simulink model "P2_SIL_Model_Diag"  (R2016a)
settings: Solver=ode2  StartTime=0.0  StopTime=Cycle_End  RelTol=1e-3
undefined symbols (not defined in the file): air, APP1_OOR, APP2_OOR, APP_Conversion_IN, APP_Mismatch, bms_inletair_temp, bms_maxchargecurrent, bms_maxdischargecurrent, BMS_Notfallkuehlung, BPP_Flt, cal, clt, ClutchEngag, CrankRequest, dcdc, eng, Engine, EngOverTemp, ENGTRQ_MSMCH_Degraded_CP, ENGTRQ_MSMCH_ErrCritical_CP, ENGTRQ_MSMCH_LimpHome_CP, EngTrqMismatch, env, ess, ESS, ESSOverTemp, fd, FFD, g, gb, Grade, IMG, KeyPos_Flt, KeyPosition, lib_APP_Conversion_IN, lib_ESS_plant_V1_2, lib_OBC_Manager, LossCAN, max_vehicle_rad_air_flow, MCUOverTemp, mot, MotDirMismatch, MotOverTemp, MotTrqMismatch, mph2kph, mph2ms, NeutralGear, obc, OBC_Manager, ParkGear, PRNDL_Flt, ReverseGear, RFD, rho, ShiftLeverPosition, sigbuilder_block, Speed, t_amb, time, tloop ... (+2)
libraries: simulink x104, EC2_libraries x12, Diagnostic x11, lib_CANerror_Detect x3, Utility x1
(part 7 of 11)

== system P2_SIL_Model_Diag/Controller/HSC/Camaro Fault Detection/Signal Generator /BMS_Signals ==
  BMS_rollingAliveCnt : Subsystem
  Bus Creator : BusCreator  Inputs=9
  Constant{1..8} (8 alike) : Constant
  tag scope: BMS_Signals=global
  wires:
  Constant7/1 -> Bus Creator/4  "BMS_hvBusVolt_V"
  Bus Creator/1 -> [BMS_Signals]  "BMS_Signals"
  Constant2/1 -> Bus Creator/3  "BMS_essTemp_K"
  Constant1/1 -> Bus Creator/2  "BMS_hvBattVolt_V"
  Constant3/1 -> Bus Creator/5  "BMS_closeContactorsCmd"
  Constant4/1 -> Bus Creator/6  "BMS_contactorsClsd"
  Constant5/1 -> Bus Creator/7  "BMS_essCurr_A"
  Constant6/1 -> Bus Creator/8  "BMS_essSOC_0_1"
  Constant8/1 -> Bus Creator/9  "BMS_gdf"
  BMS_rollingAliveCnt/1(Out1) -> Bus Creator/1

== system P2_SIL_Model_Diag/Controller/HSC/Camaro Fault Detection/Signal Generator /Clutch_Signals ==
  note: LvrPosTrnsShft
      | TransEstGear
      | LockupCmd
  note: TransEstGear
      | 0 : Not Supported
      | 1 : First Gear
      | 2 : Second Gear
      | 3 : Third Gear
      | 4 : Fourth Gear
      | 5 : Fifth Gear
      | 6 : Sixth Gear
      | 7 : Seventh Gear
      | 8 : Eight Gear
      | 10: EVT Mode 1
      | 11: EVT Mode 2
      | 12: CVT Forward Gear
      | 13: Neutral Gear
      | 14: Reverse Gear
      | 15: Park Gear
  note: Lever Position:
      | 1 P
      | 2 R
      | 3 N
      | 4 D
      |
      | 1 clutch lock-up
      | 0 clutch unlock
  Bus Creator : BusCreator  Inputs=3
  Clutch_Rolling : Subsystem
  Constant : Constant
  Constant2 : Constant
  tag scope: Clutch_Signals=global
  wires:
  Constant2/1 -> Bus Creator/3  "clt_plant_spd_out"
  Constant/1 -> Bus Creator/2  "Engage_Clutch"
  Bus Creator/1 -> [Clutch_Signals]  "Clutch_Signals"
  Clutch_Rolling/1(Out1) -> Bus Creator/1

== system P2_SIL_Model_Diag/Controller/HSC/Camaro Fault Detection/Signal Generator /Driver_Signals ==
  Bus Creator1 : BusCreator  Inputs=6
  Constant{1..6} (6 alike) : Constant
  tag scope: Driver_Signals=global
  wires:
  Bus Creator1/1 -> [Driver_Signals]  "Driver_Signals"
  Constant4/1 -> Bus Creator1/2  "BPP%"
  Constant5/1 -> Bus Creator1/3  "keyPos"
  Constant3/1 -> Bus Creator1/1  "APP1%"
  Constant6/1 -> Bus Creator1/4  "APP2%"
  Constant1/1 -> Bus Creator1/5  "PRNDL"
  Constant2/1 -> Bus Creator1/6  "V [mph]"

== system P2_SIL_Model_Diag/Controller/HSC/Camaro Fault Detection/Signal Generator /ECM_Signals ==
  Bus Creator : BusCreator  Inputs=6
  Constant{1..4} (4 alike) : Constant
  ECM_CAN_Rolling : Subsystem
  EngBrkTrq[Nm] : Constant
  tag scope: ECM_Signals=global
  wires:
  Constant1/1 -> Bus Creator/2  "ECMTrqCmd[Nm]"
  Bus Creator/1 -> [ECM_Signals]  "ECM_Signals"
  Constant2/1 -> Bus Creator/3  "Engine_Speed[rpm]"
  Constant3/1 -> Bus Creator/4  "Engine_Temp[DegC]"
  Constant4/1 -> Bus Creator/5  "EngRunAtv_0_1"
  EngBrkTrq[Nm]/1 -> Bus Creator/6  "EngActStdyStTorq_Nm"
  ECM_CAN_Rolling/1(Out1) -> Bus Creator/1

== system P2_SIL_Model_Diag/Controller/HSC/Camaro Fault Detection/Signal Generator /MCU_Signals ==
  note: From sensor
  note: From sensor
  note: From sensor
  note: From HSC
  note: From Sensor
  note: Note: motor direction feedback from HSC
  note: Torque_Command from HSC
  Bus Creator : BusCreator  Inputs=10
  Constant{1..7,9..10} (9 alike) : Constant
  MCU_CAN_rolling : Subsystem
  tag scope: MCU_Signals=global
  wires:
  Constant1/1 -> Bus Creator/2  "MCUTemp_degC"
  Bus Creator/1 -> [MCU_Signals]  "MCU_Signals"
  Constant2/1 -> Bus Creator/3  "Motor_Temp_degC"
  Constant3/1 -> Bus Creator/4  "MCUTrqCmd[Nm]"
  Constant4/1 -> Bus Creator/6  "Motor_Speed[rpm]"
  Constant5/1 -> Bus Creator/7  "Direction_Command_01"
  Constant6/1 -> Bus Creator/5  "Torque_Feedback[Nm]"
  Constant7/1 -> Bus Creator/8  "Direction_Feedback"
  Constant9/1 -> Bus Creator/9  "Inverter_Enable_State"
  Constant10/1 -> Bus Creator/10  "DC_Bus_Voltage"
  MCU_CAN_rolling/1(Out1) -> Bus Creator/1

== system P2_SIL_Model_Diag/Controller/HSC/Camaro Fault Detection/Signal Generator /TCM_Signals ==
  note: Lever Position:
      | 1 P
      | 2 R
      | 3 N
      | 4 D
      |
      | 1 clutch lock-up
      | 0 clutch unlock
  note: TransEstGear calculated in TCM
      | 0 : Not Supported
      | 1 : First Gear
      | 2 : Second Gear
      | 3 : Third Gear
      | 4 : Fourth Gear
      | 5 : Fifth Gear
      | 6 : Sixth Gear
      | 7 : Seventh Gear
      | 8 : Eight Gear
      | 10: EVT Mode 1
      | 11: EVT Mode 2
      | 12: CVT Forward Gear
      | 13: Neutral Gear
      | 14: Reverse Gear
      | 15: Park Gear
  note: LvrPosTrnsShft ==PRNDL
      | TransEstGear
      | LockupCmd
  Bus Creator : BusCreator  Inputs=4
  Constant : Constant
  Constant1 : Constant
  Constant2 : Constant
  TCM_Rolling : Subsystem
  tag scope: TCM_Signals=global
  wires:
  Bus Creator/1 -> [TCM_Signals]  "TCM_Signals"
  Constant/1 -> Bus Creator/2  "LvrPosTrnsShft"
  Constant1/1 -> Bus Creator/3  "TransEstGear"
  Constant2/1 -> Bus Creator/4  "LockupCmd"
  TCM_Rolling/1(Out1) -> Bus Creator/1

== system P2_SIL_Model_Diag/Controller/HSC/Camaro Fault Detection/SystemDiag/Combined_SystemDiagnostics ==
  note: Combined_Powertrain: System Diagnostics
  In1 : Inport
  Bus Creator : BusCreator  Inputs=1
  Bus Selector : BusSelector  OutputSignals=Driver_Input_Status.Driver_Input_Status,BMS_Status.BMS_Status,MCU_Status.MCU_Status,ECM_Status.ECM_Status,TCM_CompDiag.TCM_Status,Clutch_Status.Clutch_Status
  Combined_System_Diagnostics : Stateflow chart  TreatAsAtomicUnit=on
  Override Combined_System Status : Subsystem  AncestorBlock=Diagnostic/Camaro Diagnostic/Input Conversions/DriverInput_Conversions/Override APP (%)
  Out1 : Outport
  wires:
  In1/1 -> Bus Selector/1
  Bus Creator/1 -> Out1/1  "Combined_SystemDiagOut"
  Override Combined_System Status/1(Out1) -> Bus Creator/1  "Combined_SystemStatus"
  Bus Selector/1 -> Combined_System_Diagnostics/1(Driver_Input_Status)  "<Driver_Input_Status>"
  Bus Selector/2 -> Combined_System_Diagnostics/2(BMS_Status)  "<BMS_Status>"
  Bus Selector/3 -> Combined_System_Diagnostics/3(MCU_Status)  "<MCU_Status>"
  Bus Selector/4 -> Combined_System_Diagnostics/4(ECM_Status)  "<ECM_Status>"
  Bus Selector/5 -> Combined_System_Diagnostics/5(TCM_Status)  "<TCM_Status>"
  Bus Selector/6 -> Combined_System_Diagnostics/6(Clutch_Status)  "<Clutch_Status>"
  Combined_System_Diagnostics/1(Combined_SystemStatus) -> Override Combined_System Status/1(In1)

== system P2_SIL_Model_Diag/Controller/HSC/Camaro Fault Detection/SystemDiag/eSystemDiagnostics ==
  note: BMS_Status:
      | Offline: 0
      | Limited: 1
      | Online: 2
      |
      | MCU_Status
      | Offline: 0
      | Limited: 1
      | Online :2
  note: 0: SystemStatus: Offline
      | 1: SystemStatus Limited
      | 2: SystemStatus Online
  note: eSystem: System Diagnostics
  In1 : Inport
  Bus Creator : BusCreator  Inputs=1
  Bus Selector : BusSelector  OutputSignals=BMS_Status,MCU_Status,Driver_Input_Status,TCM_Status
  Override eSystem Status : Subsystem  AncestorBlock=Diagnostic/Camaro Diagnostic/Input Conversions/DriverInput_Conversions/Override APP (%)
  To Workspace2 : ToWorkspace  VariableName=eSystemStatus  SaveFormat=Timeseries  SampleTime=-1
  eSystem_Diagnostics : Stateflow chart  TreatAsAtomicUnit=on
  Out1 : Outport
  wires:
  In1/1 -> Bus Selector/1
  Bus Selector/1 -> eSystem_Diagnostics/1(BMS_Status)  "<BMS_Status>"
  Bus Selector/2 -> eSystem_Diagnostics/2(MCU_Status)  "<MCU_Status>"
  Bus Creator/1 -> Out1/1  "eSystemDiagOut"
  Bus Selector/3 -> eSystem_Diagnostics/3(Driver_Input_Status)  "<Driver_Input_Status>"
  Override eSystem Status/1(Out1) -> To Workspace2/1, Bus Creator/1  "eSystemStatus"
  eSystem_Diagnostics/1(eSystemStatus) -> Override eSystem Status/1(In1)
  Bus Selector/4 -> eSystem_Diagnostics/4(TCM_Status)  "<TCM_Status>"

== system P2_SIL_Model_Diag/Controller/HSC/Camaro Fault Detection/SystemDiag/iceSystemDiagnostics ==
  note: iceSystem: System Diagnostics
  In1 : Inport
  Bus Creator : BusCreator  Inputs=1
  Bus Selector : BusSelector  OutputSignals=ECM_Status,Clutch_Status,TCM_Status,Driver_Input_Status
  Override iceSystem Status : Subsystem  AncestorBlock=Diagnostic/Camaro Diagnostic/Input Conversions/DriverInput_Conversions/Override APP (%)
  To Workspace2 : ToWorkspace  VariableName=iceSystemStatus  SaveFormat=Timeseries  SampleTime=-1
  iceSystem_Diagnostics : Stateflow chart  TreatAsAtomicUnit=on
  Out1 : Outport
  wires:
  Override iceSystem Status/1(Out1) -> To Workspace2/1, Bus Creator/1  "iceSystemStatus"
  Bus Selector/1 -> iceSystem_Diagnostics/1(ECM_Status)  "<ECM_Status>"
  Bus Creator/1 -> Out1/1  "iceSystemDiagOut"
  In1/1 -> Bus Selector/1
  Bus Selector/3 -> iceSystem_Diagnostics/3(TCM_Status)  "<TCM_Status>"
  Bus Selector/4 -> iceSystem_Diagnostics/4(Driver_Input_Status)  "<Driver_Input_Status>"
  iceSystem_Diagnostics/1(iceSystemStatus) -> Override iceSystem Status/1(In1)
  Bus Selector/2 -> iceSystem_Diagnostics/2(Clutch_Status)  "<Clutch_Status>"

== system P2_SIL_Model_Diag/Controller/HSC/Driver_Requests/APP_BPP to DrvIntndAxlTrq1/Post Driver Intnded Axle Torque ==
  APP : Inport
  TransGearRatio : Inport  Port=2
  Mode : Inport  Port=3
  Compare To Constant1 : simulink/Logic and Bit Operations/Compare To Constant  relop=>=  const=2  OutDataTypeStr=boolean
  Constant : Constant  Value=eng.plant.trq_max_hot_point  VectorParams1D=off
  Constant1 : Constant  Value=FFD.Ratio
  Constant2 : Constant  Value=mot.plant.init.motor.trq_max.points.trq  VectorParams1D=off
  Constant3 : Constant  Value=RFD.Ratio
  Gain1 : Gain  Gain=1/100
  Gain2 : Gain  Gain=1/100
  Lookup Table : Lookup  InputValues="[0 10  100]"  Table="[0 0  100]"  LookUpMeth=Interpolation-Use End Values
  Product : Product  Inputs=4  RndMeth=Zero
  Product1 : Product  Inputs=3  RndMeth=Zero
  Ratio Filter : Subsystem
  Switch3 : Switch  Threshold=1
  DrvIntndAxlTrq : Outport
  wires:
  Lookup Table/1 -> Gain2/1, Gain1/1
  Mode/1 -> Compare To Constant1/1
  Product1/1 -> Switch3/3
  Constant2/1 -> Product1/1
  Gain2/1 -> Product1/2
  Constant3/1 -> Product1/3  "ratio"
  Switch3/1 -> DrvIntndAxlTrq/1
  TransGearRatio/1 -> Ratio Filter/1(Ratio)
  Compare To Constant1/1 -> Switch3/2
  Product/1 -> Switch3/1
  APP/1 -> Lookup Table/1
  Constant/1 -> Product/1
  Gain1/1 -> Product/2
  Constant1/1 -> Product/3  "ratio"
  Ratio Filter/1(Filtered_Ratio) -> Product/4

== system P2_SIL_Model_Diag/Controller/HSC/Driver_Requests/APP_BPP to DrvIntndAxlTrq2/Post Driver Intnded Axle Torque ==
  note: //*Missing logic for Engine Only Mode*//
  note: //*If mode==2 (CS Mode - Engine Drive) OR mode==4 (Sports Mode) pass Mot trq+Eng Trq
      | If mode==1 (CD Mode) or mode==3 (CS Mode-Motor Drive) pass MotTrq*//
  APP : Inport
  TransGearRatio : Inport  Port=2
  Mode : Inport  Port=3
  Bus Creator : BusCreator  Inputs=1
  Compare To Constant1 : simulink/Logic and Bit Operations/Compare To Constant  relop===  const=2  OutDataTypeStr=boolean
  Compare To Constant2 : simulink/Logic and Bit Operations/Compare To Constant  relop===  const=4  OutDataTypeStr=boolean
  Constant : Constant  Value=eng.plant.trq_max_hot_point  VectorParams1D=off
  Constant1 : Constant  Value=fd.plant.init.ratio
  Constant2 : Constant  Value=mot.plant.init.motor.trq_max.points.trq  VectorParams1D=off
  Constant3 : Constant  Value=mot.plant.init.motor.trq_max.points.trq  VectorParams1D=off
  Gain1 : Gain  Gain=1/100
  Gain2 : Gain  Gain=1/100
  Logical Operator : Logic  Operator=OR  AllPortsSameDT=off  OutDataTypeStr=boolean
  Lookup Table : Lookup  Commented=on  InputValues="[0 10  100]"  Table="[0 0  100]"  LookUpMeth=Interpolation-Use End Values
  Memory : Memory
  Product : Product  RndMeth=Zero
  Product1 : Product  RndMeth=Zero
  Product2 : Product  Inputs=3  RndMeth=Zero
  Ratio Filter : Subsystem
  Sum1 : Sum
  Switch3 : Switch  Threshold=1
  Terminator : Terminator  Commented=on
  DrvIntndAxlTrq : Outport
  tag scope: DrvIntdAxleTrq=global
  wires:
  Ratio Filter/1(Filtered_Ratio) -> Product2/2
  Constant1/1 -> Product2/3  "ratio"
  Gain1/1 -> Product/2
  Product/1 -> Switch3/1
  Switch3/1 -> Product2/1  "DrvIntndAxlTrq"
  Gain2/1 -> Product1/2
  Constant2/1 -> Product1/1
  Product1/1 -> Switch3/3
  Mode/1 -> Memory/1
  Bus Creator/1 -> DrvIntndAxlTrq/1
  TransGearRatio/1 -> Ratio Filter/1(Ratio)
  Product2/1 -> [DrvIntdAxleTrq], Bus Creator/1  "DrvIntndAxlTrq"
  Memory/1 -> Compare To Constant2/1, Compare To Constant1/1
  Constant/1 -> Sum1/2
  Sum1/1 -> Product/1
  APP/1 -> Gain2/1, Gain1/1
  Constant3/1 -> Sum1/1
  Compare To Constant1/1 -> Logical Operator/1
  Compare To Constant2/1 -> Logical Operator/2
  Logical Operator/1 -> Switch3/2

== system P2_SIL_Model_Diag/Controller/HSC/Driver_Requests/Vehicle_Shutdown/Components Disabled ==
  Sensors : Inport
  Diagnostics : Inport  Port=2
  Bus Selector : BusSelector  OutputSignals=from_CAN.fromEBCAN.from_ECM.EngActStdyStTorq,from_CAN.fromEBCAN.from_ECM.EngSpd_RPM,from_CAN.fromVEH_CAN.from_TCM.TransEstGear
  Bus Selector1 : BusSelector  OutputSignals=HV_Diagnostics.HVShtDwnCmpltd
  Compare To Constant1 : simulink/Logic and Bit Operations/Compare To Constant  relop===  const=ParkGear  OutDataTypeStr=boolean
  Compare To Constant2 : simulink/Logic and Bit Operations/Compare To Constant  relop=<=  const=1  OutDataTypeStr=boolean
  Compare To Constant3 : simulink/Logic and Bit Operations/Compare To Constant  relop=<=  const=1  OutDataTypeStr=boolean
  Compare To Constant4 : simulink/Logic and Bit Operations/Compare To Constant  relop===  const=ReverseGear  OutDataTypeStr=boolean
  Latch : EC2_libraries/Latch
  Logical Operator1 : Logic  Inputs=3  AllPortsSameDT=off  OutDataTypeStr=boolean
  Logical Operator2 : Logic  AllPortsSameDT=off  OutDataTypeStr=boolean
  Comp_Disabled : Outport
  wires:
  Compare To Constant4/1 -> Latch/2
  Latch/1 -> Logical Operator1/2
  Compare To Constant3/1 -> Logical Operator2/2
  Compare To Constant2/1 -> Logical Operator2/1
  Bus Selector/2 -> Compare To Constant3/1  "<EngSpd_RPM>"
  Bus Selector/1 -> Compare To Constant2/1  "<EngActStdyStTorq>"
  Logical Operator1/1 -> Comp_Disabled/1  "Components_Disabled"
  Bus Selector/3 -> Compare To Constant4/1, Compare To Constant1/1  "<TransEstGear>"
  Sensors/1 -> Bus Selector/1
  Logical Operator2/1 -> Logical Operator1/1
  Compare To Constant1/1 -> Latch/1  "ParkGearOn"
  Diagnostics/1 -> Bus Selector1/1
  Bus Selector1/1 -> Logical Operator1/3  "<HVShtDwnCmpltd>"

== system P2_SIL_Model_Diag/Controller/HSC/Driver_Requests/Vehicle_Startup/Enable Propulsion ==
  Sensors : Inport
  Bus Creator : BusCreator  Inputs=2
  Bus Selector : BusSelector  OutputSignals=from_CAN.fromVEH_CAN.from_BCM.BrkPdlPos,from_CAN.fromVEH_CAN.from_TCM.TransEstGear,from_CAN.fromVEH_CAN.from_BCM.SysPwrMd
  CTC1 : simulink/Logic and Bit Operations/Compare To Constant  relop=<  const=2  OutDataTypeStr=boolean
  CTC2 : simulink/Logic and Bit Operations/Compare To Constant  relop=>  const=2  OutDataTypeStr=boolean
  CTC4 : simulink/Logic and Bit Operations/Compare To Constant  relop===  const=ParkGear  OutDataTypeStr=uint8
  CTC5 : simulink/Logic and Bit Operations/Compare To Constant  relop=>  const=0  OutDataTypeStr=uint8
  Latch : EC2_libraries/Latch
  Logical Operator1 : Logic  Operator=OR  AllPortsSameDT=off  OutDataTypeStr=boolean
  Logical Operator2 : Logic  Inputs=3  AllPortsSameDT=off  OutDataTypeStr=boolean
  StartVehEnable : Outport
  EnablePrplsnStatus : Outport  Port=2
  wires:
  CTC2/1 -> Logical Operator2/3
  Bus Selector/2 -> CTC4/1  "<TransEstGear>"
  Sensors/1 -> Bus Selector/1
  Bus Selector/1 -> CTC5/1  "<BrkPdlPos>"
  CTC4/1 -> Logical Operator2/2
  CTC5/1 -> Logical Operator2/1
  Logical Operator2/1 -> Bus Creator/1, Logical Operator1/1, Latch/1  "NormalStart"
  Latch/1 -> Bus Creator/2, Logical Operator1/2  "AutoStart"
  CTC1/1 -> Latch/2
  Bus Selector/3 -> CTC2/1, CTC1/1  "<SysPwrMd>"
  Bus Creator/1 -> EnablePrplsnStatus/1
  Logical Operator1/1 -> StartVehEnable/1  "Start Enabled"

== system P2_SIL_Model_Diag/Controller/HSC/Powertrain Manager/HV Manager/APM_Manager ==
  HV_Status : Inport
  Sensors : Inport  Port=2
  Bus Creator1 : BusCreator  Inputs=1
  Bus Creator2 : BusCreator  Inputs=4
  Bus Selector1 : BusSelector  OutputSignals=from_CAN.fromHV_CAN.from_APM.Accessory_Pwr_Mod_Gen_Status_1.APMLwVltOtptCrntUns
  Bus Selector2 : BusSelector  OutputSignals=ReadyToCharge,ReadyToDrive
  Compare To Constant2 : simulink/Logic and Bit Operations/Compare To Constant  relop=<  const=cal.apm.MaxShtdwnCurrent  OutDataTypeStr=uint8
  Constant6 : Constant  Value=0
  Constant9 : Constant  Value=cal.apm.LowVoltageSetpoint
  Data Type Conversion : DataTypeConversion
  Logical Operator : Logic  AllPortsSameDT=off  OutDataTypeStr=boolean
  Logical Operator1 : Logic  Operator=OR  AllPortsSameDT=off  OutDataTypeStr=boolean
  Logical Operator3 : Logic  Operator=NOT  AllPortsSameDT=off  OutDataTypeStr=boolean
  APM Controls : Outport
  APM Status : Outport  Port=2
  wires:
  Constant6/1 -> Bus Creator2/4  "HybContClrLgsDiag"
  Constant9/1 -> Bus Creator2/3  "LwVltStpntCmnd"
  Data Type Conversion/1 -> Logical Operator3/1, Bus Creator2/2  "LowVoltEnblRq"
  Logical Operator1/1 -> Data Type Conversion/1, Bus Creator2/1  "PrplsnSysAtv"
  Logical Operator/1 -> Bus Creator1/1  "APM_ShtdwnRdy"
  Compare To Constant2/1 -> Logical Operator/2
  Bus Selector2/2 -> Logical Operator1/2  "<ReadyToDrive>"
  Bus Selector2/1 -> Logical Operator1/1  "<ReadyToCharge>"
  Sensors/1 -> Bus Selector1/1
  HV_Status/1 -> Bus Selector2/1
  Bus Creator2/1 -> APM Controls/1
  Logical Operator3/1 -> Logical Operator/1
  Bus Creator1/1 -> APM Status/1
  Bus Selector1/1 -> Compare To Constant2/1  "<APMLwVltOtptCrntUns>"

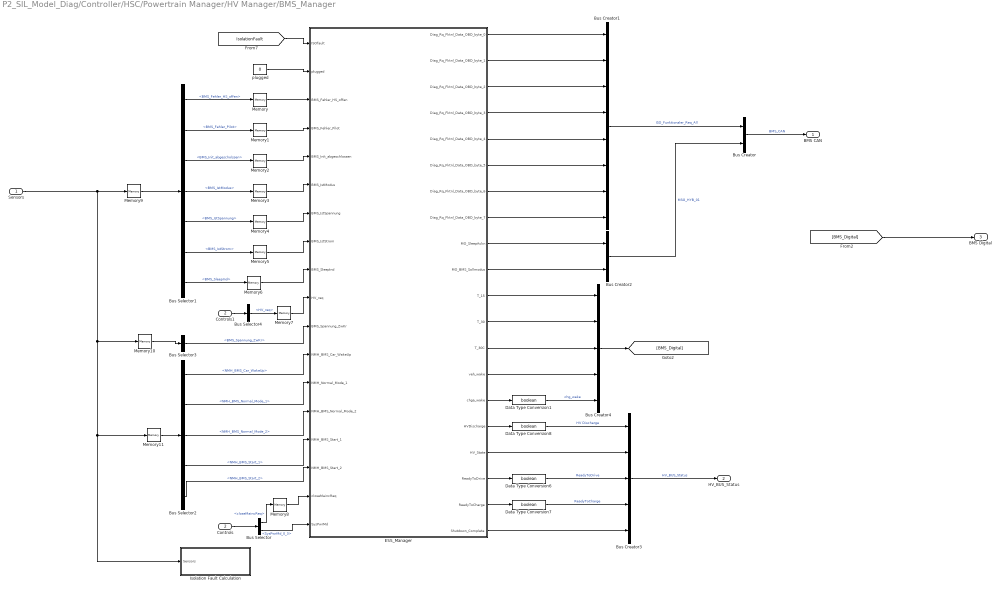
== system P2_SIL_Model_Diag/Controller/HSC/Powertrain Manager/HV Manager/BMS_Manager ==
  Sensors : Inport
  Controls : Inport  Port=2
  Bus Creator : BusCreator  Inputs=2
  Bus Creator1 : BusCreator  Inputs=8
  Bus Creator2 : BusCreator  Inputs=2
  Bus Creator3 : BusCreator  Inputs=5
  Bus Creator4 : BusCreator  Inputs=5
  Bus Selector : BusSelector  OutputSignals=closeMaincReq,SysPwrMd_0_3
  Bus Selector1 : BusSelector  OutputSignals=from_CAN.fromHV_CAN.from_BMSHybrid.BMS_HYB_02.BMS_Fehler_HS_offen,from_CAN.fromHV_CAN.from_BMSHybrid.BMS_HYB_02.BMS_Fehler_Pilot,from_CAN.fromHV_CAN.from_BMSHybrid.BMS_HYB_02.BMS_Init_abgescholssen,from_CAN.fromHV_CAN.from_BMSHybrid.BMS_HYB_02.BMS_IstModus,from_CAN.fromHV_CAN.from_BMSHybrid.BMS_HYB_02.BMS_IstSpannung,from_CAN.fromHV_CAN.from_BMSHybrid.BMS_HYB_02.BMS_IstStrom,from_CAN.fromHV_CAN.from_BMSHybrid.BMS_HYB_02.BMS_SleepInd
  Bus Selector2 : BusSelector  OutputSignals=from_CAN.fromEBCAN.from_BMSAntrieb.NMH_BMS.NMH_BMS_Car_WakeUp,from_CAN.fromEBCAN.from_BMSAntrieb.NMH_BMS.NMH_BMS_Normal_Mode_1,from_CAN.fromEBCAN.from_BMSAntrieb.NMH_BMS.NMH_BMS_Normal_Mode_2,from_CAN.fromEBCAN.from_BMSAntrieb.NMH_BMS.NMH_BMS_Start_1,from_CAN.fromEBCAN.from_BMSAntrieb.NMH_BMS.NMH_BMS_Start_2
  Bus Selector3 : BusSelector  OutputSignals=from_CAN.fromHV_CAN.from_BMSHybrid.BMS_Spannung_ZwKr
  Bus Selector4 : BusSelector  OutputSignals=HV_req
  Controls1 : InportShadow  Port=2
  Data Type Conversion{1,6..8} (4 alike) : DataTypeConversion  OutDataTypeStr=boolean
  ESS_Manager : Stateflow chart  TreatAsAtomicUnit=on
  Isolation Fault Calculation : Subsystem
  Memory{,1..11} (12 alike) : Memory
  plugged : Constant  Value=0
  BMS CAN : Outport
  HV_BUS_Status : Outport  Port=2
  BMS Digital : Outport  Port=3
  wires:
  Bus Selector1/1 -> Memory/1  "<BMS_Fehler_HS_offen>"
  Bus Selector1/2 -> Memory1/1  "<BMS_Fehler_Pilot>"
  Bus Selector1/3 -> Memory2/1  "<BMS_Init_abgescholssen>"
  Bus Selector1/4 -> Memory3/1  "<BMS_IstModus>"
  Bus Selector1/5 -> Memory4/1  "<BMS_IstSpannung>"
  Bus Selector1/6 -> Memory5/1  "<BMS_IstStrom>"
  Bus Selector1/7 -> Memory6/1  "<BMS_SleepInd>"
  Bus Selector4/1 -> Memory7/1  "<HV_req>"
  Bus Selector2/1 -> ESS_Manager/12(NMH_BMS_Car_WakeUp)  "<NMH_BMS_Car_WakeUp>"
  Bus Selector2/2 -> ESS_Manager/13(NMH_Normal_Mode_1)  "<NMH_BMS_Normal_Mode_1>"
  Bus Selector2/3 -> ESS_Manager/14(NMH_BMS_Normal_Mode_2)  "<NMH_BMS_Normal_Mode_2>"
  Bus Selector2/4 -> ESS_Manager/15(NMH_BMS_Start_1)  "<NMH_BMS_Start_1>"
  Bus Selector2/5 -> ESS_Manager/16(NMH_BMS_Start_2)  "<NMH_BMS_Start_2>"
  Bus Selector3/1 -> ESS_Manager/11(BMS_Spannung_ZwKr)  "<BMS_Spannung_ZwKr>"
  plugged/1 -> ESS_Manager/2(plugged)
  ESS_Manager/1(Diag_Rq_Fktnl_Data_OBD_byte_0) -> Bus Creator1/1
  ESS_Manager/2(Diag_Rq_Fktnl_Data_OBD_byte_1) -> Bus Creator1/2
  ESS_Manager/3(Diag_Rq_Fktnl_Data_OBD_byte_2) -> Bus Creator1/3
  ESS_Manager/4(Diag_Rq_Fktnl_Data_OBD_byte_3) -> Bus Creator1/4
  ESS_Manager/5(Diag_Rq_Fktnl_Data_OBD_byte_4) -> Bus Creator1/5
  ESS_Manager/6(Diag_Rq_Fktnl_Data_OBD_byte_5) -> Bus Creator1/6
  ESS_Manager/7(Diag_Rq_Fktnl_Data_OBD_byte_6) -> Bus Creator1/7
  ESS_Manager/8(Diag_Rq_Fktnl_Data_OBD_byte_7) -> Bus Creator1/8
  ESS_Manager/9(MO_SleepAckn) -> Bus Creator2/1
  ESS_Manager/10(MO_BMS_Sollmodus) -> Bus Creator2/2
  ESS_Manager/11(T_15) -> Bus Creator4/1
  Data Type Conversion6/1 -> Bus Creator3/3  "ReadyToDrive"
  Data Type Conversion7/1 -> Bus Creator3/4  "ReadyToCharge"
  Data Type Conversion8/1 -> Bus Creator3/1  "HV Discharge"
  Bus Creator2/1 -> Bus Creator/2  "MSG_HYB_01"
  Bus Creator1/1 -> Bus Creator/1  "ISO_Funktionaler_Req_All"
  [IsolationFault] -> ESS_Manager/1(ISOfault)
  Sensors/1 -> Memory11/1, Isolation Fault Calculation/1(Sensors), Memory10/1, Memory9/1
  ESS_Manager/16(HVDischarge) -> Data Type Conversion8/1
  ESS_Manager/18(ReadyToDrive) -> Data Type Conversion6/1
  ESS_Manager/19(ReadyToCharge) -> Data Type Conversion7/1
  ESS_Manager/20(Shutdown_Complete) -> Bus Creator3/5
  ESS_Manager/12(T_30) -> Bus Creator4/2
  ESS_Manager/15(chga_wake) -> Data Type Conversion1/1
  ESS_Manager/13(T_30C) -> Bus Creator4/3
  ESS_Manager/14(veh_wake) -> Bus Creator4/4
  ESS_Manager/17(HV_State) -> Bus Creator3/2
  Bus Creator3/1 -> HV_BUS_Status/1  "HV_BUS_Status"
  Controls/1 -> Bus Selector/1
  Bus Selector/1 -> Memory8/1  "<closeMaincReq>"
  Controls1/1 -> Bus Selector4/1
  Bus Creator/1 -> BMS CAN/1  "BMS_CAN"
  Bus Creator4/1 -> [BMS_Digital]
  [BMS_Digital] -> BMS Digital/1
  Data Type Conversion1/1 -> Bus Creator4/5  "chg_wake"
  Memory/1 -> ESS_Manager/3(BMS_Fehler_HS_offen)
  Memory1/1 -> ESS_Manager/4(BMS_Fehler_Pilot)
  Memory2/1 -> ESS_Manager/5(BMS_Init_abgeschlossen)
  Memory3/1 -> ESS_Manager/6(BMS_IstModus)
  Memory4/1 -> ESS_Manager/7(BMS_IstSpannung)
  Memory5/1 -> ESS_Manager/8(BMS_IstStrom)
  Memory6/1 -> ESS_Manager/9(BMS_SleepInd)
  Memory7/1 -> ESS_Manager/10(HV_req)
  Memory8/1 -> ESS_Manager/17(closeMaincReq)
  Memory9/1 -> Bus Selector1/1
  Memory11/1 -> Bus Selector2/1
  Memory10/1 -> Bus Selector3/1
  Bus Selector/2 -> ESS_Manager/18(SysPwrMd)  "<SysPwrMd_0_3>"

== system P2_SIL_Model_Diag/Controller/HSC/Powertrain Manager/HV Manager/OBC_Manager ==
  note: $Author: eo1000 $
      | $Rev: 508 $
      | $Date: 2014-01-12 12:42:33 -0500 (Sun, 12 Jan 2014) $
  HV_Status : Inport
  Sensors : Inport  Port=2
  Bus Creator1 : BusCreator  Inputs=6
  Bus Creator3 : BusCreator  Inputs=3
  Bus Selector1 : BusSelector  OutputSignals=from_CAN.fromHV_CAN.from_OBC.NLG5_ST.NLG5_S_UM_II,from_CAN.fromHV_CAN.from_OBC.NLG5_ACT_I.NLG5_OC_ACT
  Bus Selector2 : BusSelector  OutputSignals=ReadyToCharge
  Compare To Constant : simulink/Logic and Bit Operations/Compare To Constant  relop===  const=0  OutDataTypeStr=boolean
  Compare To Constant1 : simulink/Logic and Bit Operations/Compare To Constant  relop=<  const=cal.obc.MaxShtdwnCurrent  OutDataTypeStr=boolean
  Constant1 : Constant  Value=0
  Constant10 : Constant  Value=cal.obc.MaxChargeCurrent_Level2
  Constant11 : Constant  Value=cal.obc.MaxChargeCurrent_Level1
  Constant12 : Constant  Value=0
  Constant4 : Constant  Value=0
  Constant5 : Constant  Value=cal.obc.MaxMainsCurrent
  Constant6 : Constant  Value=cal.obc.MaxOutputVoltage
  Data Type Conversion1 : DataTypeConversion
  Data Type Conversion2 : DataTypeConversion
  EVSE_chgReady : Constant
  Latch1 : EC2_libraries/Latch
  Logical Operator : Logic  Operator=OR  AllPortsSameDT=off  OutDataTypeStr=boolean
  MinMax1 : MinMax  Inputs=2
  Switch : Switch  Criteria=u2 > Threshold
  Switch2 : Switch  Criteria=u2 > Threshold
  chg_done : Constant
  OBC CAN : Outport
  OBC Status : Outport  Port=2
  wires:
  HV_Status/1 -> Bus Selector2/1
  Constant6/1 -> Bus Creator1/5  "NLG5_OV_COM"
  Constant5/1 -> Bus Creator1/4  "NLG5_MC_MAX"
  Latch1/1 -> Bus Creator1/3  "NLG5_C_C_EN"
  Constant1/1 -> Bus Creator1/2  "NLG5_C_C_EL"
  Constant4/1 -> Bus Creator1/1  "NLG5_C_CP_V"
  Sensors/1 -> Bus Selector1/1
  Bus Creator1/1 -> OBC CAN/1  "OBC_Controls"
  Bus Selector2/1 -> Latch1/1  "<ReadyToCharge>"
  Switch2/1 -> Bus Creator1/6  "NLG5_OC_COM"
  Constant10/1 -> Switch/1
  Constant11/1 -> Switch/3
  Switch/1 -> MinMax1/2, Bus Creator3/2  "EVSELmtdChgCrnt"
  Constant12/1 -> Switch2/1
  MinMax1/1 -> Switch2/3, Bus Creator3/1  "LmtdOBCChgCrnt"
  Logical Operator/1 -> Data Type Conversion2/1
  Compare To Constant/1 -> Logical Operator/2
  Data Type Conversion1/1 -> Switch/2
  Data Type Conversion2/1 -> Switch2/2
  Compare To Constant1/1 -> Latch1/2, Bus Creator3/3  "OBC_ShtdwnRdy"
  Bus Creator3/1 -> OBC Status/1  "OBC_Status"
  Bus Selector1/2 -> Compare To Constant1/1  "<NLG5_OC_ACT>"
  Bus Selector1/1 -> Data Type Conversion1/1  "<NLG5_S_UM_II>"
  chg_done/1 -> Logical Operator/1
  EVSE_chgReady/1 -> Compare To Constant/1

== system P2_SIL_Model_Diag/Controller/HSC/Powertrain Manager/PowertrainSUSD/Crank Engine ==
  note: TransEstGear
      | $0=Not Supported
      | $1=First Gear
      | $2=Second Gear
      | $3=Third Gear
      | $4=Fourth Gear
      | $5=Fifth Gear
      | $6=Sixth Gear
      | $7=Seventh Gear
      | $8=Eighth Gear
      | $A=EVT Mode 1
      | $B=EVT Mode 2
      | $C=CVT Forward Gear
      | $D=Neutral Gear
      | $E=Reverse Gear
      | $F=Park Gear
  note: EngState:
      | Init: EngState = 0;
      | Crank_Engine: EngState = 1;
      | Crank_Disable: EngState = 2;
      | StopEngCmd: EngState = 3;
      | StopEngComplete: EngState = 4;
      | Eng will not Crank: EngState = -1;
  note: Key Position
      | KeyOFF: 0
      | KeyAccessory: 1
      | KeyIgnition: 2
      | KeyCrank = 3
  Sensors : Inport
  Control : Inport  Port=2
  Bus Creator2 : BusCreator  Inputs=2
  Bus Selector : BusSelector  OutputSignals=from_CAN.fromEBCAN.from_ECM.EngRunAtv
  Bus Selector1 : BusSelector  OutputSignals=SysPwrMd_0_3,ClutchEngage,EnablePrplsn
  CS_FSwitch : Constant  Value=0
  Constant : Constant  Value=cal.Time.CrankEngine
  Constant1 : Constant  Value=CrankRequest
  Constant2 : Constant  Value=CrankRequest
  Crank_Stop_Engine : Stateflow chart  TreatAsAtomicUnit=on
  Data Type Conversion1 : DataTypeConversion
  Data Type Conversion2 : DataTypeConversion  OutDataTypeStr=boolean
  Gain1 : Gain  Gain=1/tloop
  Switch : Switch  Criteria=u2 > Threshold
  Switch1 : Switch  Criteria=u2 > Threshold
  Upper Limit : EC2_libraries/Upper Limit  Uplimit=2
  EngStatus : Outport
  EngCrankCmd : Outport  Port=2
  SysPwrMdOut : Outport  Port=3
  wires:
  Bus Creator2/1 -> EngStatus/1
  Crank_Stop_Engine/2(EngState) -> Bus Creator2/2  "EngState"
  Constant2/1 -> Switch1/1
  Switch1/1 -> Crank_Stop_Engine/1(SysPwrMd), Bus Creator2/1, Upper Limit/1  "SysPwrMd_Switched"
  Gain1/1 -> Crank_Stop_Engine/5(CrankEngTime)
  Sensors/1 -> Bus Selector/1
  Bus Selector1/3 -> Data Type Conversion2/1  "<EnablePrplsn>"
  Bus Selector/1 -> Data Type Conversion1/1  "<EngRunAtv>"
  Constant/1 -> Gain1/1
  Data Type Conversion1/1 -> Crank_Stop_Engine/4(EngRunAtv)
  Switch/1 -> SysPwrMdOut/1
  Crank_Stop_Engine/1(CrankCmd) -> EngCrankCmd/1, Switch/2
  Upper Limit/1 -> Switch/3
  Constant1/1 -> Switch/1
  Control/1 -> Bus Selector1/1
  Bus Selector1/1 -> Switch1/3  "<SysPwrMd_0_3>"
  Bus Selector1/2 -> Crank_Stop_Engine/2(ClutchEngage)  "<ClutchEngage>"
  CS_FSwitch/1 -> Switch1/2
  Data Type Conversion2/1 -> Crank_Stop_Engine/3(EnablePrplsn)

== system P2_SIL_Model_Diag/Controller/HSC/Powertrain Manager/Torque Distribution/AxlTrq_to_EngTrq1 ==
  note: //From engine axle torque to engine torque//
  In1 : Inport
  Compare To Constant : simulink/Logic and Bit Operations/Compare To Constant  relop===  const=0  OutDataTypeStr=boolean
  Constant1 : Constant  Value=max(gb.plant.init.ratio.map)
  Constant5 : Constant  Value=fd.plant.init.ratio
  Divide1 : Product  Inputs=*//
  Rate Limiter : RateLimiter  RisingSlewLimit=Engine.trq_uprate  FallingSlewLimit=Engine.trq_derate  SampleTimeMode=inherited
  Ratio Filter : Subsystem
  Switch : Switch  Criteria=u2 > Threshold
  Out1 : Outport
  wires:
  Ratio Filter/1(Filtered_Ratio) -> Compare To Constant/1, Switch/3
  Rate Limiter/1 -> Out1/1
  Switch/1 -> Divide1/3
  Constant1/1 -> Switch/1
  Compare To Constant/1 -> Switch/2
  [TransRatio] -> Ratio Filter/1(Ratio)
  Divide1/1 -> Rate Limiter/1
  Constant5/1 -> Divide1/2
  In1/1 -> Divide1/1

== system P2_SIL_Model_Diag/Controller/HSC/Powertrain Manager/Torque Distribution/AxlTrq_to_EngTrq2 ==
  note: //From engine axle torque to engine torque//
  In1 : Inport
  Compare To Constant : simulink/Logic and Bit Operations/Compare To Constant  relop===  const=0  OutDataTypeStr=boolean
  Constant1 : Constant  Value=max(gb.plant.init.ratio.map)
  Constant5 : Constant  Value=fd.plant.init.ratio
  Divide1 : Product  Inputs=*//
  Rate Limiter : RateLimiter  RisingSlewLimit=Engine.trq_uprate  FallingSlewLimit=Engine.trq_derate  SampleTimeMode=inherited
  Ratio Filter : Subsystem
  Switch : Switch  Criteria=u2 > Threshold
  Out1 : Outport
  wires:
  In1/1 -> Divide1/1
  Constant5/1 -> Divide1/2
  Divide1/1 -> Rate Limiter/1
  [TransRatio] -> Ratio Filter/1(Ratio)
  Compare To Constant/1 -> Switch/2
  Constant1/1 -> Switch/1
  Switch/1 -> Divide1/3
  Rate Limiter/1 -> Out1/1
  Ratio Filter/1(Filtered_Ratio) -> Switch/3, Compare To Constant/1

== system P2_SIL_Model_Diag/Controller/HSC/Powertrain Manager/Torque Distribution/AxlTrq_to_MtrTrq1 ==
  note: //From motor axle torque to motor torque//
  In1 : Inport
  Compare To Constant : simulink/Logic and Bit Operations/Compare To Constant  relop===  const=0  OutDataTypeStr=boolean
  Constant1 : Constant  Value=max(gb.plant.init.ratio.map)
  Constant5 : Constant  Value=fd.plant.init.ratio
  Divide : Product  Inputs=*//
  Rate Limiter : RateLimiter  RisingSlewLimit=mcu.plant.init.trq_uprate  FallingSlewLimit=mcu.plant.init.trq_derate  SampleTimeMode=inherited
  Ratio Filter : Subsystem
  Switch : Switch  Criteria=u2 > Threshold
  Out1 : Outport
  wires:
  Ratio Filter/1(Filtered_Ratio) -> Compare To Constant/1, Switch/3
  Switch/1 -> Divide/3
  Rate Limiter/1 -> Out1/1
  Constant1/1 -> Switch/1
  Compare To Constant/1 -> Switch/2
  [TransRatio] -> Ratio Filter/1(Ratio)
  Divide/1 -> Rate Limiter/1
  Constant5/1 -> Divide/2
  In1/1 -> Divide/1

== system P2_SIL_Model_Diag/Controller/HSC/Powertrain Manager/Torque Distribution/AxlTrq_to_MtrTrq2 ==
  note: //From motor axle torque to motor torque//
  In1 : Inport
  Compare To Constant : simulink/Logic and Bit Operations/Compare To Constant  relop===  const=0  OutDataTypeStr=boolean
  Constant1 : Constant  Value=max(gb.plant.init.ratio.map)
  Constant5 : Constant  Value=fd.plant.init.ratio
  Divide : Product  Inputs=*//
  Rate Limiter : RateLimiter  RisingSlewLimit=mcu.plant.init.trq_uprate  FallingSlewLimit=mcu.plant.init.trq_derate  SampleTimeMode=inherited
  Ratio Filter : Subsystem
  Switch : Switch  Criteria=u2 > Threshold
  Out1 : Outport
  wires:
  In1/1 -> Divide/1
  Constant5/1 -> Divide/2
  Divide/1 -> Rate Limiter/1
  [TransRatio] -> Ratio Filter/1(Ratio)
  Compare To Constant/1 -> Switch/2
  Constant1/1 -> Switch/1
  Rate Limiter/1 -> Out1/1
  Switch/1 -> Divide/3
  Ratio Filter/1(Filtered_Ratio) -> Switch/3, Compare To Constant/1

== system P2_SIL_Model_Diag/Controller/HSC/Powertrain Manager/Torque Distribution/Signal Builder1 ==
  Demux : Demux  Tag=STV Demux  Outputs=1
  FromWs : FromWorkspace  Tag=STV FromWs  VariableName=tuvar  SampleTime=0
      SigBuilderData=|
      | common.afterFinalStr = 'Extrapolate'
      | common.sampleTime = 0
      | dataSet.timeRange = [0 500]
      | dataSet.name = 'Group 1'
      | sbobj.Groups.Name = 'Group 1'
      | sbobj.Groups.Signals.Name = 'Signal 1'
      | sbobj.Groups.Signals.XData = [0 200 300 500]
      | sbobj.Groups.Signals.YData = [0 0 0 0]
      | sbobj.Groups.TimeRange = [0 500]
  Signal 1 : Outport  Tag=STV Outport
  wires:
  Demux/1 -> Signal 1/1
  FromWs/1 -> Demux/1

== system P2_SIL_Model_Diag/Controller/HSC/Powertrain Manager/Torque Distribution/Signal Builder2 ==
  Demux : Demux  Tag=STV Demux  Outputs=1
  FromWs : FromWorkspace  Tag=STV FromWs  VariableName=tuvar  SampleTime=0
      SigBuilderData=|
      | common.afterFinalStr = 'Extrapolate'
      | common.sampleTime = 0
      | dataSet.timeRange = [0 500]
      | dataSet.name = 'Group 1'
      | sbobj.Groups.Name = 'Group 1'
      | sbobj.Groups.Signals.Name = 'Signal 1'
      | sbobj.Groups.Signals.XData = [0 200 300 500]
      | sbobj.Groups.Signals.YData = [2 2 2 2]
      | sbobj.Groups.TimeRange = [0 500]
  Signal 1 : Outport  Tag=STV Outport
  wires:
  FromWs/1 -> Demux/1
  Demux/1 -> Signal 1/1

== system P2_SIL_Model_Diag/Controller/HSC/Powertrain Manager/Torque Distribution/Signal Builder3 ==
  Demux : Demux  Tag=STV Demux  Outputs=1
  FromWs : FromWorkspace  Tag=STV FromWs  VariableName=tuvar  SampleTime=0
      SigBuilderData=|
      | common.afterFinalStr = 'Extrapolate'
      | common.sampleTime = 0
      | dataSet.timeRange = [0 500]
      | dataSet.name = 'Group 1'
      | sbobj.Groups.Name = 'Group 1'
      | sbobj.Groups.Signals.Name = 'Signal 1'
      | sbobj.Groups.Signals.XData = [0 200 300 500]
      | sbobj.Groups.Signals.YData = [2 2 2 2]
      | sbobj.Groups.TimeRange = [0 500]
  Signal 1 : Outport  Tag=STV Outport
  wires:
  Demux/1 -> Signal 1/1
  FromWs/1 -> Demux/1

== system P2_SIL_Model_Diag/Controller/HSC/Powertrain Manager/Torque Distribution/Signal Builder4 ==
  Demux : Demux  Tag=STV Demux  Outputs=1
  FromWs : FromWorkspace  Tag=STV FromWs  VariableName=tuvar  SampleTime=0
      SigBuilderData=|
      | common.afterFinalStr = 'Extrapolate'
      | common.sampleTime = 0
      | dataSet.timeRange = [0 500]
      | dataSet.name = 'Group 1'
      | sbobj.Groups.Name = 'Group 1'
      | sbobj.Groups.Signals.Name = 'Signal 1'
      | sbobj.Groups.Signals.XData = [0 200 300 500]
      | sbobj.Groups.Signals.YData = [0 0 0 0]
      | sbobj.Groups.TimeRange = [0 500]
  Signal 1 : Outport  Tag=STV Outport
  wires:
  FromWs/1 -> Demux/1
  Demux/1 -> Signal 1/1

== system P2_SIL_Model_Diag/Controller/HSC/Powertrain Manager/Torque Distribution/Supervisory  Control  Logic1/VehReady.CD_Limited.MotTrqCalc1 ==
  note: //This is the available motor torque. Consider moving it do diagnostic//
  APP : Inport
  BPP : Inport  Port=2
  VehSpd : Inport  Port=3
  ShftLvrPos : Inport  Port=4
  MotSpeed : Inport  Port=5
  DrvIntdAxleTrq : Inport  Port=6
  TransRatio : Inport  Port=7
  MotTrqMismchDegraded : Inport  Port=8
  MotTrqMismchLimp : Inport  Port=9
  essTempRange : Inport  Port=10
  MCUTempRange : Inport  Port=11
  MotorTempRange : Inport  Port=12
  f : TriggerPort  TriggerType=function-call  VariantControl=Variant
      settings: CopyFcn=Stateflow.SLINSF.SimulinkMan.removeBlockPreDeleteFcn  PreDeleteFcn=Stateflow.SLINSF.SimulinkMan.unsafePredeleteFcn
  % to 1 : Gain  Gain=1/100
  "% to 1 " : Gain  Gain=1/100
  Constant : Constant  Value=0
  Constant1 : Constant  Value=0
  Constant2 : Constant  Value=fd.plant.init.ratio
  Divide : Product  Inputs=***
  Divide1 : Product  Inputs=**
  Divide2 : Product  Inputs=***
  Index Vector : MultiPortSwitch  DataPortOrder=Zero-based contiguous  Inputs=5  zeroidx=on
  MinMax : MinMax  Inputs=2
  MotSpeed1 : InportShadow  Port=5
  Motor Troque Mismatch Mitigation : Subsystem
  OverTemperature Mitigation : Subsystem
  Peak trq max - Motoring : Lookup  InputValues=mot.plant.init.regen.trq_max.idx1_spd  Table=mot.plant.init.motor.trq_max.map  LookUpMeth=Interpolation-Use End Values  SaturateOnIntegerOverflow=on
  Peak trq max - Regen : Lookup  InputValues=mot.plant.init.regen.trq_max.idx1_spd  Table=mot.plant.init.regen.trq_max.map  LookUpMeth=Interpolation-Use End Values  SaturateOnIntegerOverflow=on
  Regen Trq Derating : Lookup_n-D  NumberOfTableDimensions=1  BreakpointsForDimension1=[0 10 20 30 40]  Table=[0 0.025 0.05 0.1 1]  ExtrapMethod=Clip  UseLastTableValue=on  InternalRulePriority=Speed  RndMeth=Simplest  InputSameDT=on
  Switch : Switch  Criteria=u2 > Threshold
  limit to 200Nm : Saturate  UpperLimit=0  LowerLimit=-200
  T : Outport
  wires:
  BPP/1 -> "% to 1 "/1
  "% to 1 "/1 -> Divide/1
  Divide/1 -> limit to 200Nm/1
  VehSpd/1 -> Regen Trq Derating/1
  Regen Trq Derating/1 -> Divide/3
  % to 1/1 -> Divide1/2
  ShftLvrPos/1 -> Index Vector/1
  [TrqCalc] -> Index Vector/4  "R"
  [TrqCalc] -> Index Vector/6  "D"
  Index Vector/1 -> T/1
  Constant/1 -> Index Vector/2  "Between Ranges"
  Constant1/1 -> Index Vector/3  "P"
  [TrqCalc] -> Index Vector/5  "N"
  APP/1 -> % to 1/1, Switch/2
  MotSpeed/1 -> Peak trq max - Motoring/1  "RPM"
  Peak trq max - Motoring/1 -> Divide1/1
  Divide1/1 -> Switch/1
  MotSpeed1/1 -> Peak trq max - Regen/1  "RPM"
  Peak trq max - Regen/1 -> Divide/2
  Constant2/1 -> Divide2/1
  Switch/1 -> Divide2/2
  limit to 200Nm/1 -> Switch/3
  TransRatio/1 -> Divide2/3
  DrvIntdAxleTrq/1 -> MinMax/1  "river"
  Divide2/1 -> MinMax/2  "motor"
  MinMax/1 -> Motor Troque Mismatch Mitigation/1(In1)
  MotTrqMismchDegraded/1 -> Motor Troque Mismatch Mitigation/2(MotTrqMismchDegraded)
  MotTrqMismchLimp/1 -> Motor Troque Mismatch Mitigation/3(MotTrqMismchLimp)
  Motor Troque Mismatch Mitigation/1(Out1) -> OverTemperature Mitigation/1(In1)
  essTempRange/1 -> OverTemperature Mitigation/2(essTempRange)
  MCUTempRange/1 -> OverTemperature Mitigation/3(MCUTempRange)
  MotorTempRange/1 -> OverTemperature Mitigation/4(MotorTempRange)
  OverTemperature Mitigation/1(Out1) -> [TrqCalc]

== system P2_SIL_Model_Diag/Controller/HSC/Powertrain Manager/Torque Distribution/Supervisory  Control  Logic1/VehReady.CD_Mode.MotTrqCalc ==
  APP : Inport
  BPP : Inport  Port=2
  VehSpd : Inport  Port=3
  Shifter : Inport  Port=4
  MotSpeed : Inport  Port=5
  f : TriggerPort  TriggerType=function-call  VariantControl=Variant
      settings: CopyFcn=Stateflow.SLINSF.SimulinkMan.removeBlockPreDeleteFcn  PreDeleteFcn=Stateflow.SLINSF.SimulinkMan.unsafePredeleteFcn
  % to 1 : Gain  Gain=1/100
  "% to 1 " : Gain  Gain=1/100
  Constant : Constant  Value=0
  Constant1 : Constant  Value=0
  Divide : Product  Inputs=***
  Divide1 : Product  Inputs=**
  Index Vector : MultiPortSwitch  DataPortOrder=Zero-based contiguous  Inputs=5  zeroidx=on
  MotSpeed1 : InportShadow  Port=5
  Peak trq max - Motoring : Lookup  InputValues=mot.plant.init.regen.trq_max.idx1_spd  Table=mot.plant.init.motor.trq_max.map  LookUpMeth=Interpolation-Use End Values  SaturateOnIntegerOverflow=on
  Peak trq max - Regen : Lookup  InputValues=mot.plant.init.regen.trq_max.idx1_spd  Table=mot.plant.init.regen.trq_max.map  LookUpMeth=Interpolation-Use End Values  SaturateOnIntegerOverflow=on
  Regen Trq Derating : Lookup_n-D  NumberOfTableDimensions=1  BreakpointsForDimension1=[0 10 20 30 40]  Table=[0 0.025 0.05 0.1 1]  ExtrapMethod=Clip  UseLastTableValue=on  InternalRulePriority=Speed  RndMeth=Simplest  InputSameDT=on
  Switch : Switch  Criteria=u2 > Threshold
  limit to 200Nm : Saturate  UpperLimit=0  LowerLimit=-200
  T : Outport
  wires:
  BPP/1 -> "% to 1 "/1
  "% to 1 "/1 -> Divide/1
  Divide/1 -> limit to 200Nm/1
  VehSpd/1 -> Regen Trq Derating/1
  Regen Trq Derating/1 -> Divide/3
  % to 1/1 -> Divide1/2
  Switch/1 -> [TrqCalc]
  Shifter/1 -> Index Vector/1
  [TrqCalc] -> Index Vector/4  "R"
  [TrqCalc] -> Index Vector/6  "D"
  Index Vector/1 -> T/1
  Constant/1 -> Index Vector/2  "Between Ranges"
  Constant1/1 -> Index Vector/3  "P"
  [TrqCalc] -> Index Vector/5  "N"
  APP/1 -> % to 1/1, Switch/2
  MotSpeed/1 -> Peak trq max - Motoring/1  "RPM"
  Peak trq max - Motoring/1 -> Divide1/1
  Divide1/1 -> Switch/1
  MotSpeed1/1 -> Peak trq max - Regen/1  "RPM"
  Peak trq max - Regen/1 -> Divide/2
  limit to 200Nm/1 -> Switch/3

== system P2_SIL_Model_Diag/Controller/HSC/Powertrain Manager/Torque Distribution/Supervisory  Control  Logic1/VehReady.CD_Mode.MotTrqCalc1 ==
  note: //This is the available motor torque. Consider moving it do diagnostic//
  APP : Inport
  BPP : Inport  Port=2
  VehSpd : Inport  Port=3
  ShftLvrPos : Inport  Port=4
  MotSpeed : Inport  Port=5
  DrvIntdAxleTrq : Inport  Port=6
  TransRatio : Inport  Port=7
  eSystemStatus : Inport  Port=8
  f : TriggerPort  TriggerType=function-call  VariantControl=Variant
      settings: CopyFcn=Stateflow.SLINSF.SimulinkMan.removeBlockPreDeleteFcn  PreDeleteFcn=Stateflow.SLINSF.SimulinkMan.unsafePredeleteFcn
  % to 1 : Gain  Gain=1/100
  "% to 1 " : Gain  Gain=1/100
  Compare To Zero : simulink/Logic and Bit Operations/Compare To Zero  relop===  OutDataTypeStr=boolean
  Constant : Constant  Value=0
  Constant1 : Constant  Value=0
  Constant2 : Constant  Value=fd.plant.init.ratio
  Constant3 : Constant  Value=0
  Divide : Product  Inputs=***
  Divide1 : Product  Inputs=**
  Divide2 : Product  Inputs=***
  Index Vector : MultiPortSwitch  DataPortOrder=Zero-based contiguous  Inputs=5  zeroidx=on
  MinMax : MinMax  Inputs=2
  MotSpeed1 : InportShadow  Port=5
  Peak trq max - Motoring : Lookup  InputValues=mot.plant.init.regen.trq_max.idx1_spd  Table=mot.plant.init.motor.trq_max.map  LookUpMeth=Interpolation-Use End Values  SaturateOnIntegerOverflow=on
  Peak trq max - Regen : Lookup  InputValues=mot.plant.init.regen.trq_max.idx1_spd  Table=mot.plant.init.regen.trq_max.map  LookUpMeth=Interpolation-Use End Values  SaturateOnIntegerOverflow=on
  Regen Trq Derating : Lookup_n-D  NumberOfTableDimensions=1  BreakpointsForDimension1=[0 10 20 30 40]  Table=[0 0.025 0.05 0.1 1]  ExtrapMethod=Clip  UseLastTableValue=on  InternalRulePriority=Speed  RndMeth=Simplest  InputSameDT=on
  Switch : Switch  Criteria=u2 > Threshold
  Switch1 : Switch  Threshold=1
  limit to 200Nm : Saturate  UpperLimit=0  LowerLimit=-200
  T : Outport
  wires:
  BPP/1 -> "% to 1 "/1
  "% to 1 "/1 -> Divide/1
  Divide/1 -> limit to 200Nm/1
  VehSpd/1 -> Regen Trq Derating/1
  Regen Trq Derating/1 -> Divide/3
  % to 1/1 -> Divide1/2
  ShftLvrPos/1 -> Index Vector/1
  [TrqCalc] -> Index Vector/4  "R"
  [TrqCalc] -> Index Vector/6  "D"
  Index Vector/1 -> T/1
  Constant/1 -> Index Vector/2  "Between Ranges"
  Constant1/1 -> Index Vector/3  "P"
  [TrqCalc] -> Index Vector/5  "N"
  APP/1 -> % to 1/1, Switch/2
  MotSpeed/1 -> Peak trq max - Motoring/1  "RPM"
  Peak trq max - Motoring/1 -> Divide1/1
  Divide1/1 -> Switch/1
  MotSpeed1/1 -> Peak trq max - Regen/1  "RPM"
  Peak trq max - Regen/1 -> Divide/2
  Constant2/1 -> Divide2/1
  Switch/1 -> Divide2/2
  limit to 200Nm/1 -> Switch/3
  TransRatio/1 -> Divide2/3
  DrvIntdAxleTrq/1 -> MinMax/1  "river"
  Divide2/1 -> MinMax/2  "motor"
  MinMax/1 -> Switch1/3
  Switch1/1 -> [TrqCalc]
  eSystemStatus/1 -> Compare To Zero/1
  Compare To Zero/1 -> Switch1/2
  Constant3/1 -> Switch1/1

== system P2_SIL_Model_Diag/Controller/HSC/Powertrain Manager/Torque Distribution/Supervisory  Control  Logic1/VehReady.CS_Mode.Engine_Drive.ChgCalc ==
  EngSpeed : Inport
  APP : Inport  Port=2
  VehSpd : Inport  Port=3
  DrvIntdAxleTrq : Inport  Port=4
  TransRatio : Inport  Port=5
  f : TriggerPort  TriggerType=function-call  VariantControl=Variant
      settings: CopyFcn=Stateflow.SLINSF.SimulinkMan.removeBlockPreDeleteFcn  PreDeleteFcn=Stateflow.SLINSF.SimulinkMan.unsafePredeleteFcn
  APP Derating : Lookup_n-D  NumberOfTableDimensions=1  BreakpointsForDimension1=[0 1 2 3]  Table=[0 0 0.1 1]  ExtrapMethod=Clip  UseLastTableValue=on  InternalRulePriority=Speed  RndMeth=Simplest  InputSameDT=on
  Constant1 : Constant  Value=Engine.IdleSpeed
  Constant3 : Constant  Value=fd.plant.init.ratio
  Divide : Product  Inputs=***
  Divide2 : Product  Inputs=***
  EngOptmTrq : Lookup_n-D  NumberOfTableDimensions=1  BreakpointsForDimension1=[1550 1650 1850 2050 2350 2650 2950 3150 3250 3350]  Table="[154.020912669576\t173.623574282068\t180.662367834043\t186.327738253926\t182.858870786433\t180.175407273844\t178.037732950256\t181.891363533595\t190.985931710274\t199.537540592824]"  ExtrapMethod=Clip  UseLastTableValue=on  InternalRulePriority=Speed  RndMeth=Simplest  InputSameDT=on
  EngOptmTrq1 : Lookup_n-D  NumberOfTableDimensions=1  BreakpointsForDimension1=[1550 1650 1850 2050 2350 2650 2950 3150 3250 3350]  Table="[154.020912669576\t173.623574282068\t180.662367834043\t186.327738253926\t182.858870786433\t180.175407273844\t178.037732950256\t181.891363533595\t190.985931710274\t199.537540592824]"  ExtrapMethod=Clip  UseLastTableValue=on  InternalRulePriority=Speed  RndMeth=Simplest  InputSameDT=on
  MinMax : MinMax  Inputs=2
  Sum : Sum  Inputs=+-
  Switch : Switch  Criteria=u2 > Threshold  Threshold=Engine.IdleSpeed
  VehSpd Derating : Lookup_n-D  NumberOfTableDimensions=1  BreakpointsForDimension1=[0 5 10 20]  Table=[0 0 0.1 1]  ExtrapMethod=Clip  UseLastTableValue=on  InternalRulePriority=Speed  RndMeth=Simplest  InputSameDT=on
  Chg : Outport
  wires:
  EngSpeed/1 -> EngOptmTrq/1
  APP/1 -> APP Derating/1
  EngOptmTrq/1 -> Divide/1
  APP Derating/1 -> Divide/2
  VehSpd/1 -> VehSpd Derating/1
  VehSpd Derating/1 -> Divide/3
  Constant3/1 -> Divide2/1
  Divide/1 -> Divide2/2
  Divide2/1 -> Sum/1  "engine"
  TransRatio/1 -> Divide2/3
  DrvIntdAxleTrq/1 -> Sum/2  "driver"
  MinMax/1 -> Switch/3
  EngOptmTrq1/1 -> MinMax/2
  Constant1/1 -> EngOptmTrq1/1
  Sum/1 -> Chg/1
